simulink model "NonLinear"  (R2024b)
settings: Solver=ode45  StartTime=0.0  StopTime=T  RelTol=1e-3
InitFcn:
  | leminscate;
StopFcn:
  | plottingNonLinear;
values from neighbouring files (symbols this model uses):
  Ts = 0.01    [leminscate.m]
libraries: robotmobilelib x1
settings Model: Creator=salva  LastModifiedBy=salva

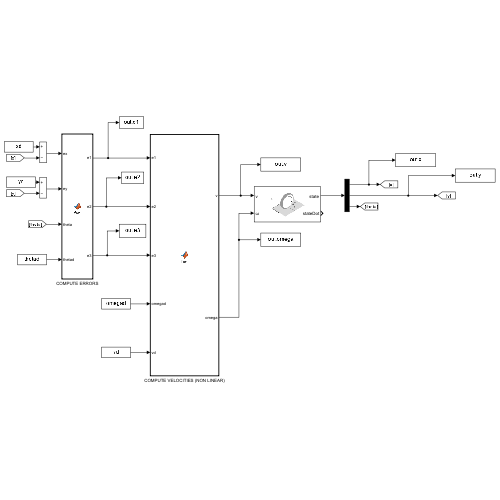
[thumbnail: Simulink's stored preview of the top-level diagram]
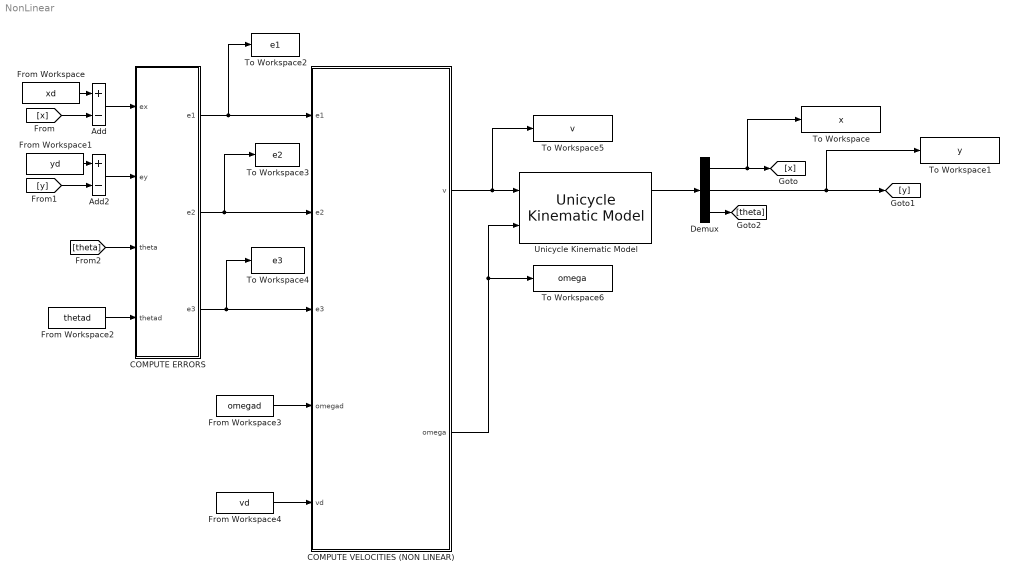
== system NonLinear ==
  Add : Sum  Inputs=+-
  Add2 : Sum  Inputs=+-
  COMPUTE ERRORS : MATLAB Function  TreatAsAtomicUnit=on
  COMPUTE VELOCITIES (NON LINEAR) : MATLAB Function  TreatAsAtomicUnit=on
  Demux : Demux  Outputs=3
  From Workspace : FromWorkspace  VariableName=xd
  From Workspace1 : FromWorkspace  VariableName=yd
  From Workspace2 : FromWorkspace  VariableName=thetad
  From Workspace3 : FromWorkspace  VariableName=omegad
  From Workspace4 : FromWorkspace  VariableName=vd
  To Workspace : ToWorkspace  VariableName=x  SaveFormat=Timeseries  SampleTime=Ts
  To Workspace1 : ToWorkspace  VariableName=y  SaveFormat=Timeseries  SampleTime=Ts
  To Workspace2 : ToWorkspace  VariableName=e1  SaveFormat=Timeseries  SampleTime=Ts
  To Workspace3 : ToWorkspace  VariableName=e2  SaveFormat=Timeseries  SampleTime=Ts
  To Workspace4 : ToWorkspace  VariableName=e3  SaveFormat=Timeseries  SampleTime=Ts
  To Workspace5 : ToWorkspace  VariableName=v  SaveFormat=Timeseries  SampleTime=Ts
  To Workspace6 : ToWorkspace  VariableName=omega  SaveFormat=Timeseries  SampleTime=Ts
  Unicycle Kinematic Model : robotmobilelib/Unicycle Kinematic Model  VehicleInputs=Vehicle Speed & Heading Angular Velocity  WheelRadius=R  WheelSpeedRange=[-Inf,Inf]  InitialState=qi  SimulateUsing=Interpreted execution
  wires:
  COMPUTE ERRORS/2(e2) -> To Workspace3/1, COMPUTE VELOCITIES (NON LINEAR)/2(e2)
  COMPUTE ERRORS/3(e3) -> To Workspace4/1, COMPUTE VELOCITIES (NON LINEAR)/3(e3)
  COMPUTE ERRORS/1(e1) -> To Workspace2/1, COMPUTE VELOCITIES (NON LINEAR)/1(e1)
  COMPUTE VELOCITIES (NON LINEAR)/1(v) -> To Workspace5/1, Unicycle Kinematic Model/1
  COMPUTE VELOCITIES (NON LINEAR)/2(omega) -> Unicycle Kinematic Model/2, To Workspace6/1
  Add/1 -> COMPUTE ERRORS/1(ex)
  From Workspace/1 -> Add/1
  [theta] -> COMPUTE ERRORS/3(theta)
  Add2/1 -> COMPUTE ERRORS/2(ey)
  From Workspace3/1 -> COMPUTE VELOCITIES (NON LINEAR)/4(omegad)
  From Workspace1/1 -> Add2/1
  Demux/2 -> To Workspace1/1, [y]
  [x] -> Add/2
  [y] -> Add2/2
  Demux/3 -> [theta]
  From Workspace2/1 -> COMPUTE ERRORS/4(thetad)
  Demux/1 -> To Workspace/1, [x]
  From Workspace4/1 -> COMPUTE VELOCITIES (NON LINEAR)/5(vd)
  Unicycle Kinematic Model/1 -> Demux/1

== matlab function NonLinear/COMPUTE VELOCITIES (NON LINEAR) ==
  data: e1 input; v output; e2 input; e3 input; omegad input; vd input; omega output
function [v,omega] = fcn(e1,e2,e3,omegad,vd)

    k1=35*vd^2+0.1*omegad^2;
    k3=40*vd^2+0.1*omegad^2;
  
    k2=90;

   
    u1=-k1*e1;
    u2=-k2*vd*(sinc(e3))*e2-k3*e3;

   
    v=vd*cos(e3)-u1;
    omega=omegad-u2;
end

== matlab function NonLinear/COMPUTE ERRORS ==
  data: ex input; e1 output; ey input; theta input; e2 output; e3 output; thetad input
function [e1,e2,e3] = fcn(ex,ey,theta,thetad)

    T=[cos(theta),sin(theta),0;
        -sin(theta),cos(theta),0;
        0,0,1];
    
    res=T*[ex;ey;thetad-theta];
    
    e1=res(1);
    e2=res(2);
    e3=res(3);

end
